simulink model "Events_2"  (Simulink 5.0)
settings: Solver=FixedStepDiscrete  StartTime=0.0  StopTime=10.0  RelTol=1e-3
settings Model: Creator=sofronis  LastModifiedBy=sofronis  ExtModeAutoUpdateStatusClock=off  AlgebraicLoopMsg=error

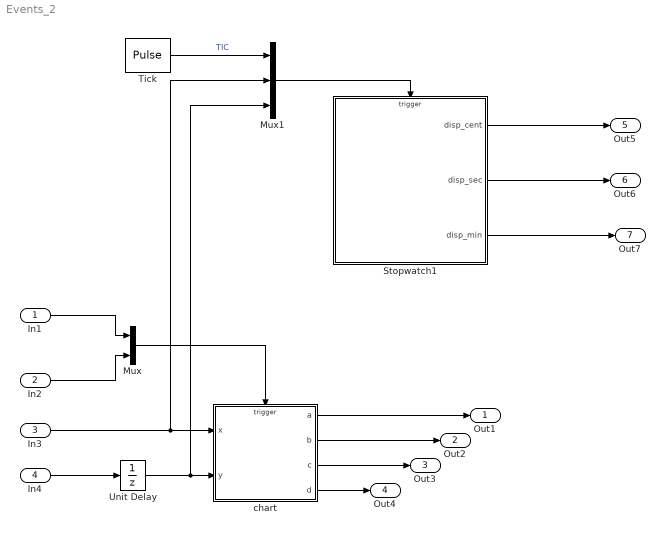
== system Events_2 ==
  In1 : Inport  SampleTime=1
  In2 : Inport  Port=2  SampleTime=1
  In3 : Inport  Port=3  SampleTime=1
  In4 : Inport  Port=4  SampleTime=1
  Mux : Mux  Inputs=2
  Mux1 : Mux  Inputs=3
  Stopwatch1 : Stateflow chart
  Tick : DiscretePulseGenerator  VectorParams1D=off
  Unit Delay : UnitDelay  SampleTime=-1
  chart : Stateflow chart
  Out1 : Outport
  Out2 : Outport  Port=2
  Out3 : Outport  Port=3
  Out4 : Outport  Port=4
  Out5 : Outport  Port=5
  Out6 : Outport  Port=6
  Out7 : Outport  Port=7
  wires:
  In1/1 -> Mux/1
  In2/1 -> Mux/2
  In3/1 -> chart/1(x), Mux1/2
  Mux/1 -> chart/Trigger
  chart/1(a) -> Out1/1
  chart/2(b) -> Out2/1
  chart/3(c) -> Out3/1
  chart/4(d) -> Out4/1
  In4/1 -> Unit Delay/1
  Unit Delay/1 -> chart/2(y), Mux1/3
  Stopwatch1/1(disp_cent) -> Out5/1
  Stopwatch1/2(disp_sec) -> Out6/1
  Tick/1 -> Mux1/1  "TIC"
  Mux1/1 -> Stopwatch1/Trigger
  Stopwatch1/3(disp_min) -> Out7/1

== stateflow chart Stopwatch1 ==
  state Stopwatch
    state Stop
      state Reset/
        en: runlap=1;
        on LAP:
        cent=0; sec=0; min=0;
        disp_cent=0; disp_sec=0;
        disp_min=0;
      state Lap_stop/
        en: runlap=2;
      (default) -> Reset : [runlap==1]
      (default) -> Lap_stop : [runlap==2]
      Lap_stop -> Reset : LAP
    state Run
      state Tick [parallel]
        state A
        (default) -> A
        A -> (junction 13) : TIC{cent++;}
        (junction 13) -> (junction 14) : [cent==100]{cent=0; sec++;}
        (junction 13) -> (junction 15)
        (junction 14) -> (junction 15)
        (junction 14) -> (junction 15) : [sec==60]{sec=0; min++;}
      state Watch [parallel]
        state Running/
          en: runlap=1;
          du:
          disp_cent=cent;
          disp_sec=sec;
          disp_min=min;
        state Lap/
          en: runlap=2;
        Running -> Lap : LAP
        Lap -> Running : LAP
        (default) -> Running : [runlap==1]
        (default) -> Lap : [runlap==2]
    Stop -> Run : START
    Run -> Stop : START
    (default) -> Stop : {runlap=1;}
  (default) -> Stopwatch
  data: runlap local int32 =1; cent local int32; sec local int32; min local int32; disp_cent output int32; disp_sec output int32; disp_min output int32
  events: TIC input EITHER_EDGE_EVENT; LAP input EITHER_EDGE_EVENT; START input EITHER_EDGE_EVENT

== stateflow chart chart ==
  state B [parallel]
    state Ba/
      en:b=x+3
    state Bb/
      en:b=x+4+y
    (default) -> Ba
    Bb -> Ba : R1/R2
    Ba -> Bb : S1/S2
  state A [parallel]
    state Aa/
      en:a=x+1
    state Ab/
      en:a=x+2
    (default) -> Aa
    Aa -> Ab : S/S1
    Ab -> Aa : R/R1
  state D [parallel]
    state Da/
      en:d=x+7
    state Db/
      en:d=x+8
    Db -> Da : R3
    (default) -> Da
    Da -> Db : S3
  state C [parallel]
    state Cb/
      en:c=x+6
    state Ca/
      en:c=x+5
    Ca -> Cb : S2/S3
    Cb -> Ca : R2/R3
    (default) -> Ca
  data: a output int32; x input int32; b output int32; c output int32; d output int32; y input int32
  events: R1 local EITHER_EDGE_EVENT; S1 local EITHER_EDGE_EVENT; R input RISING_EDGE_EVENT; S input FALLING_EDGE_EVENT; R2 local EITHER_EDGE_EVENT; S2 local EITHER_EDGE_EVENT; S3 local EITHER_EDGE_EVENT; R3 local EITHER_EDGE_EVENT
